simulink model "model_2D_2"  (R2021b)
settings: Solver=VariableStepAuto  StartTime=0.0  StopTime=discretization_time  RelTol=1e-3
settings Model: Creator=filip  LastModifiedBy=filip

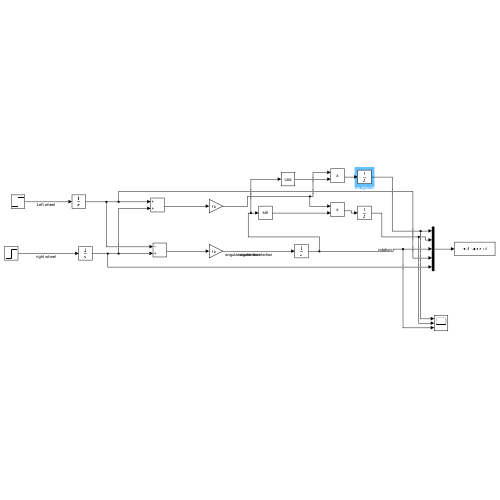
[thumbnail: Simulink's stored preview of the top-level diagram]
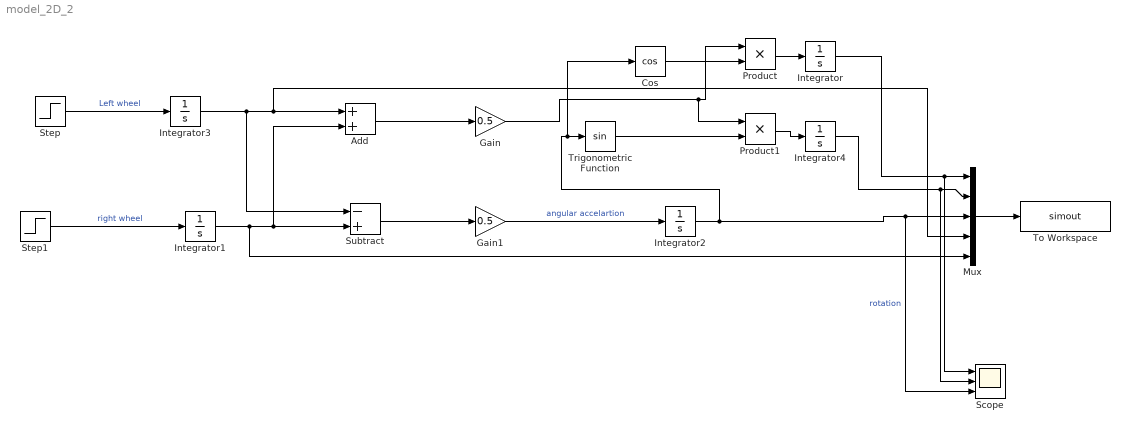
== system model_2D_2 ==
  Add : Sum
  Cos : Trigonometry  Operator=cos
  Gain : Gain  Gain=0.5
  Gain1 : Gain  Gain=0.5
  Integrator{,1..4} (5 alike) : Integrator
  Mux : Mux  Inputs=5
  Product : Product
  Product1 : Product
  Scope : Scope  NumInputPorts=3
  Step : Step  SampleTime=0
  Step1 : Step  SampleTime=0
  Subtract : Sum  Inputs=-+
  To Workspace : ToWorkspace  VariableName=simout  SaveFormat=Timeseries  SampleTime=-1
  Trigonometric Function : Trigonometry
  wires:
  Step/1 -> Integrator3/1  "Left wheel"
  Step1/1 -> Integrator1/1  "right wheel"
  Add/1 -> Gain/1
  Subtract/1 -> Gain1/1
  Gain1/1 -> Integrator2/1  "angular accelartion"
  Mux/1 -> To Workspace/1
  Integrator2/1 -> Scope/3, Mux/3, Cos/1, Trigonometric Function/1  "rotation"
  Integrator/1 -> Scope/1, Mux/1
  Integrator4/1 -> Scope/2, Mux/2
  Product/1 -> Integrator/1
  Product1/1 -> Integrator4/1
  Trigonometric Function/1 -> Product1/2
  Cos/1 -> Product/2
  Gain/1 -> Product1/1, Product/1
  Integrator3/1 -> Subtract/1, Mux/4, Add/1
  Integrator1/1 -> Mux/5, Subtract/2, Add/2
